simulink model "MagLev_Simscape"  (R2025b)
settings: Solver=VariableStepAuto  StartTime=0.0  StopTime=10.0  RelTol=1e-3
undefined symbols (not defined in the file): b_mech, g, K_force, Kd_x_dummy, Ki_i_dummy, Kp_i_dummy, Kp_x_dummy, m, R_coil, R_eff, Vsup
libraries: fl_lib x12, nesl_utility x7
settings Model: Creator=lucia  LastModifiedBy=lucianbracy
settings DebuggingCC: AlgebraicLoopMsg=none

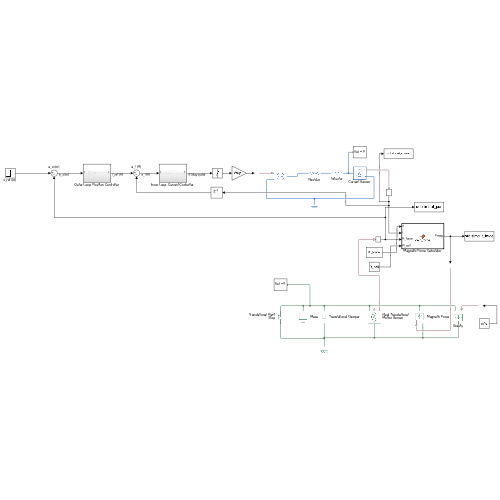
[thumbnail: Simulink's stored preview of the top-level diagram]
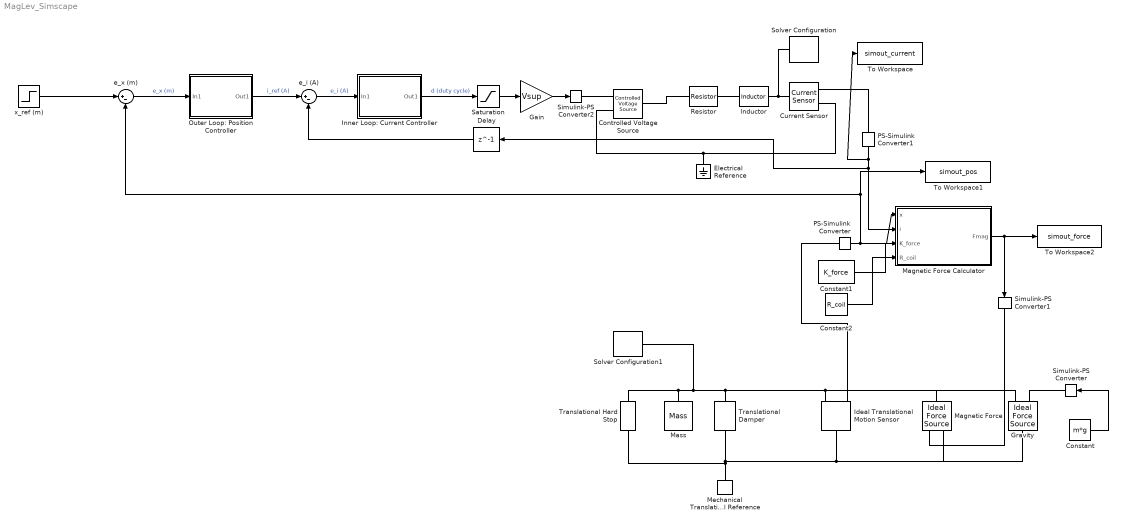
== system MagLev_Simscape ==
  Constant : Constant  Value=m*g
  Constant1 : Constant  Value=K_force
  Constant2 : Constant  Value=R_coil
  Controlled Voltage Source : fl_lib/Electrical/Electrical Sources/Controlled Voltage Source
  Current Sensor : fl_lib/Electrical/Electrical Sensors/Current Sensor
  Delay : Delay  DelayLength=1  InitialCondition=0
  Electrical Reference : fl_lib/Electrical/Electrical Elements/Electrical Reference
  Gain : Gain  Gain=Vsup
  Gravity : fl_lib/Mechanical/Mechanical Sources/Ideal Force Source
  Ideal Translational Motion Sensor : fl_lib/Mechanical/Mechanical Sensors/Ideal Translational Motion Sensor  reference=foundation.enum.MeasurementReference.difference  acceleration_port=false  velocity_port=true  position_port=true  offset=0.0254 m
  Inductor : fl_lib/Electrical/Electrical Elements/Inductor  l=L H  r=0 Ohm  g=1e-9 1/Ohm  i_specify=off  i_priority=None  i=0 A  i_nominal_specify=off  i_nominal_value=1  i_nominal_unit=A  v_specify=off  v_priority=None  v=0 V  v_nominal_specify=off  v_nominal_value=1  v_nominal_unit=V  i_L_specify=off  i_L_priority=High  i_L=0 A  i_L_nominal_specify=off  i_L_nominal_value=1  i_L_nominal_unit=A
  "Inner Loop: Current Controller " : Subsystem
  Magnetic Force : fl_lib/Mechanical/Mechanical Sources/Ideal Force Source
  Magnetic Force Calculator : MATLAB Function  TreatAsAtomicUnit=on
  Mass : fl_lib/Mechanical/Translational Elements/Mass  mass=m kg  num_ports=foundation.enum.numPorts2.one  v_specify=off  v_priority=High  v=0 m/s  v_nominal_specify=off  v_nominal_value=1  v_nominal_unit=m/s  f_specify=off  f_priority=None  f=0 N  f_nominal_specify=off  f_nominal_value=1  f_nominal_unit=N
  Mechanical Translational Reference : fl_lib/Mechanical/Translational Elements/Mechanical Translational Reference
  Outer Loop: Position Controller : Subsystem
  PS-Simulink Converter : nesl_utility/PS-Simulink Converter  PhysicalDomain=network_engine_domain  SubClassName=ps_output  LeftPortType=input  RightPortType=output  PseudoPeriodic=off  Frequencies=[]  VectorFormat=inherit  Unit=inherit  AffineConversion=off
  PS-Simulink Converter1 : nesl_utility/PS-Simulink Converter  PhysicalDomain=network_engine_domain  SubClassName=ps_output  LeftPortType=input  RightPortType=output  PseudoPeriodic=off  Frequencies=[]  VectorFormat=inherit  Unit=inherit  AffineConversion=off
  Resistor : fl_lib/Electrical/Electrical Elements/Resistor  R=R_eff Ohm  i_specify=off  i_priority=None  i=0 A  i_nominal_specify=off  i_nominal_value=1  i_nominal_unit=A  v_specify=off  v_priority=None  v=0 V  v_nominal_specify=off  v_nominal_value=1  v_nominal_unit=V
  Saturation : Saturate  UpperLimit=1  LowerLimit=0
  Simulink-PS Converter : nesl_utility/Simulink-PS Converter  PhysicalDomain=network_engine_domain  SubClassName=ps_input  LeftPortType=input  RightPortType=output  PseudoPeriodic=off  Frequencies=[]  NoiseDistribution=none  NoiseParameters=[]  Unit=1  AffineConversion=off  FilteringAndDerivatives=provide  SimscapeFilterOrder=1  InputFilterTimeConstant=0.001  UdotUserProvided=0
  Simulink-PS Converter1 : nesl_utility/Simulink-PS Converter  PhysicalDomain=network_engine_domain  SubClassName=ps_input  LeftPortType=input  RightPortType=output  PseudoPeriodic=off  Frequencies=[]  NoiseDistribution=none  NoiseParameters=[]  Unit=1  AffineConversion=off  FilteringAndDerivatives=provide  SimscapeFilterOrder=1  InputFilterTimeConstant=0.001  UdotUserProvided=0
  Simulink-PS Converter2 : nesl_utility/Simulink-PS Converter  PhysicalDomain=network_engine_domain  SubClassName=ps_input  LeftPortType=input  RightPortType=output  PseudoPeriodic=off  Frequencies=[]  NoiseDistribution=none  NoiseParameters=[]  Unit=1  AffineConversion=off  FilteringAndDerivatives=provide  SimscapeFilterOrder=1  InputFilterTimeConstant=0.001  UdotUserProvided=0
  Solver Configuration : nesl_utility/Solver Configuration  PhysicalDomain=network_engine_domain  SubClassName=solver  LeftPortType=input  RightPortType=generic  Tones=[]  Harmonics=[]  SimulateNoise=off  Profile=off  UseLocalSampling=off  EnableSwitchedLinearOptims=on  FrequencyDomain=off  UseCCode=off  RelTol=0.001  AbsTol=0.001  MinStep=1e-09  ToWorkspace=off  RevertToSquareIcSolve=off  NumHomotopyIterations=100  PhasorMode=off  PhasorModeNumHarmonics=1  ConsistencySolver=NEWTON_XTOL_AFTER_FTOL  IndexReductionMethod=DerivativeReplacement  DoDC=off  ResidualTolerance=1e-09  ConsistencyTolSource=GLOBAL  ConsistencyAbsTol=0.001  ConsistencyRelTol=0.001  ConsistencyTolFactor=0.001  UseLocalSolver=off  LocalSolverChoice=NE_BACKWARD_EULER_ADVANCER  ResolveIndetEquations=on  FunctionEvalNumThread=1  LocalSolverSampleTime=0.001  DoFixedCost=off  MaxNonlinIter=3  MaxModeIter=2  ComputeImpulses=off  ImpulseIterations=2  LinearAlgebra=auto  LinearAlgebraNumThread=0  EquationFormulation=NE_TIME_EF  DelaysMemoryBudget=1024  AutomaticFiltering=on  FilteringTimeConstant=0.001  PartitionStorageMethod=AS_NEEDED  PartitionMemoryBudget=1024  PartitionMethod=ROBUST  MultibodyUseLocalSolver=off  MultibodyLocalSolverChoice=ODE1  MultibodyLocalSolverSampleTime=0.001
  Solver Configuration1 : nesl_utility/Solver Configuration  PhysicalDomain=network_engine_domain  SubClassName=solver  LeftPortType=input  RightPortType=generic  Tones=[]  Harmonics=[]  SimulateNoise=off  Profile=off  UseLocalSampling=off  EnableSwitchedLinearOptims=on  FrequencyDomain=off  UseCCode=off  RelTol=0.001  AbsTol=0.001  MinStep=1e-09  ToWorkspace=off  RevertToSquareIcSolve=off  NumHomotopyIterations=100  PhasorMode=off  PhasorModeNumHarmonics=1  ConsistencySolver=NEWTON_XTOL_AFTER_FTOL  IndexReductionMethod=DerivativeReplacement  DoDC=off  ResidualTolerance=1e-09  ConsistencyTolSource=GLOBAL  ConsistencyAbsTol=0.001  ConsistencyRelTol=0.001  ConsistencyTolFactor=0.001  UseLocalSolver=off  LocalSolverChoice=NE_BACKWARD_EULER_ADVANCER  ResolveIndetEquations=on  FunctionEvalNumThread=1  LocalSolverSampleTime=0.001  DoFixedCost=off  MaxNonlinIter=3  MaxModeIter=2  ComputeImpulses=off  ImpulseIterations=2  LinearAlgebra=auto  LinearAlgebraNumThread=0  EquationFormulation=NE_TIME_EF  DelaysMemoryBudget=1024  AutomaticFiltering=on  FilteringTimeConstant=0.001  PartitionStorageMethod=AS_NEEDED  PartitionMemoryBudget=1024  PartitionMethod=ROBUST  MultibodyUseLocalSolver=off  MultibodyLocalSolverChoice=ODE1  MultibodyLocalSolverSampleTime=0.001
  To Workspace : ToWorkspace  VariableName=simout_current  SaveFormat=Timeseries  SampleTime=-1
  To Workspace1 : ToWorkspace  VariableName=simout_pos  SaveFormat=Timeseries  SampleTime=-1
  To Workspace2 : ToWorkspace  VariableName=simout_force  SaveFormat=Timeseries  SampleTime=-1
  Translational Damper : fl_lib/Mechanical/Translational Elements/Translational Damper  D=b_mech N*s/m  v_specify=off  v_priority=None  v=0 m/s  v_nominal_specify=off  v_nominal_value=1  v_nominal_unit=m/s  f_specify=off  f_priority=None  f=0 N  f_nominal_specify=off  f_nominal_value=1  f_nominal_unit=N
  Translational Hard Stop : fl_lib/Mechanical/Translational Elements/Translational Hard Stop  upper_bnd=0.0254 m  lower_bnd=0 m  model=simscape.enum.hardstop.smooth  stiff_up=1e5 N/m  stiff_low=1e5 N/m  D_up=100 N*s/m  D_low=100 N*s/m  transition=0.1 mm  coeff_rest=0.7  v_tol=0.001 m/s  f_tol=0.001 N  v_specify=off  v_priority=None  v=0 m/s  v_nominal_specify=off  v_nominal_value=1  v_nominal_unit=m/s  f_specify=off  f_priority=None  f=0 N  f_nominal_specify=off  f_nominal_value=1  f_nominal_unit=N  x_specify=off  x_priority=High  x=0 m  x_nominal_specify=off  x_nominal_value=1  x_nominal_unit=m  M_specify=off  M_priority=None  M=0
  e_i (A) : Sum  Inputs=|+-
  e_x (m) : Sum  Inputs=|+-
  "x_ref (m) " : Step  After=0.0127  SampleTime=0
  wires:
  Constant/1 -> Simulink-PS Converter/1
  Magnetic Force Calculator/1(Fmag) -> To Workspace2/1, Simulink-PS Converter1/1
  PS-Simulink Converter/1 -> e_x (m)/2, To Workspace1/1, Magnetic Force Calculator/1(x)
  PS-Simulink Converter1/1 -> To Workspace/1, Delay/1, Magnetic Force Calculator/2(i)
  e_i (A)/1 -> "Inner Loop: Current Controller "/1(In1)  "e_i (A)"
  e_x (m)/1 -> Outer Loop: Position Controller/1(In1)  "e_x (m)"
  "x_ref (m) "/1 -> e_x (m)/1
  Outer Loop: Position Controller/1(Out1) -> e_i (A)/1  "i_ref (A)"
  "Inner Loop: Current Controller "/1(Out1) -> Saturation/1  "d (duty cycle)"
  Saturation/1 -> Gain/1
  Delay/1 -> e_i (A)/2
  Gain/1 -> Simulink-PS Converter2/1
  Constant2/1 -> Magnetic Force Calculator/4(R_coil)
  Constant1/1 -> Magnetic Force Calculator/3(K_force)
  connections:
  Inductor/LConn1 -- Resistor/RConn1
  Current Sensor/LConn1 -- Solver Configuration/RConn1 -- Inductor/RConn1
  Current Sensor/RConn2 -- Controlled Voltage Source/RConn2 -- Electrical Reference/LConn1
  Current Sensor/RConn1 -- PS-Simulink Converter1/LConn1
  Resistor/LConn1 -- Controlled Voltage Source/LConn1
  Simulink-PS Converter2/RConn1 -- Controlled Voltage Source/RConn1
  Translational Damper/RConn1 -- Ideal Translational Motion Sensor/LConn1 -- Gravity/LConn1 -- Magnetic Force/RConn2 -- Translational Hard Stop/RConn1 -- Mechanical Translational Reference/LConn1
  Mass/LConn1 -- Solver Configuration1/RConn1 -- Ideal Translational Motion Sensor/RConn1 -- Gravity/RConn2 -- Magnetic Force/LConn1 -- Translational Damper/LConn1 -- Translational Hard Stop/LConn1
  Gravity/RConn1 -- Simulink-PS Converter/RConn1
  Simulink-PS Converter1/RConn1 -- Magnetic Force/RConn1
  PS-Simulink Converter/LConn1 -- Ideal Translational Motion Sensor/RConn3

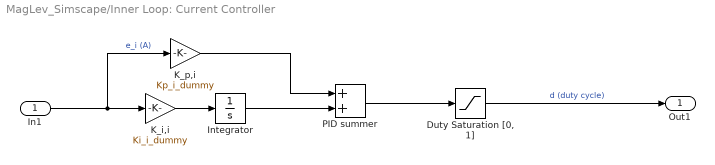
== system MagLev_Simscape/Inner Loop: Current Controller  ==
  In1 : Inport
  "Duty Saturation [0, 1]" : Saturate  UpperLimit=1  LowerLimit=0
  Integrator : Integrator
  K_i,i : Gain  Gain=Ki_i_dummy
  K_p,i : Gain  Gain=Kp_i_dummy
  PID summer : Sum
  Out1 : Outport
  wires:
  K_p,i/1 -> PID summer/1
  Integrator/1 -> PID summer/2
  "Duty Saturation [0, 1]"/1 -> Out1/1  "d (duty cycle)"
  K_i,i/1 -> Integrator/1
  In1/1 -> K_p,i/1, K_i,i/1  "e_i (A)"
  PID summer/1 -> "Duty Saturation [0, 1]"/1

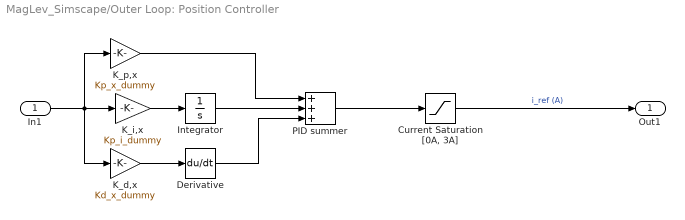
== system MagLev_Simscape/Outer Loop: Position Controller ==
  In1 : Inport
  "Current Saturation [0A, 3A]" : Saturate  UpperLimit=3  LowerLimit=0
  Derivative : Derivative
  Integrator : Integrator
  K_d,x : Gain  Gain=Kd_x_dummy
  K_i,x : Gain  Gain=Kp_i_dummy
  K_p,x : Gain  Gain=Kp_x_dummy
  PID summer : Sum  Inputs=+++
  Out1 : Outport
  wires:
  PID summer/1 -> "Current Saturation [0A, 3A]"/1
  In1/1 -> K_p,x/1, K_i,x/1, K_d,x/1
  K_i,x/1 -> Integrator/1
  K_d,x/1 -> Derivative/1
  Integrator/1 -> PID summer/2
  K_p,x/1 -> PID summer/1
  Derivative/1 -> PID summer/3
  "Current Saturation [0A, 3A]"/1 -> Out1/1  "i_ref (A)"

== matlab function MagLev_Simscape/Magnetic Force Calculator ==
  data: x input; Fmag output; i input; K_force input; R_coil input
function Fmag = calc_force(x, i, K_force, R_coil)
    x_safe = max(x, 1e-4);
    Fmag = K_force * i * x_safe / (x_safe^2 + R_coil^2)^2.5;
end
